simulink model "gm_lab2"  (R2022a)
settings: Solver=VariableStepAuto  StartTime=0.0  StopTime=5.0  RelTol=1e-3
settings Model: Creator=User  LastModifiedBy=User
settings OptimizationCC: BlockReduction=off  ConditionallyExecuteInputs=off
settings DebuggingCC: InheritedTsInSrcMsg=none

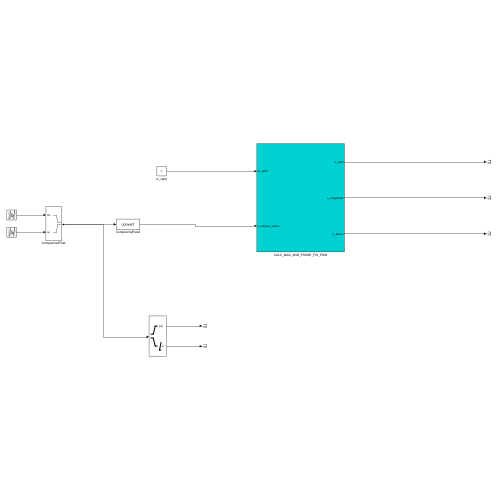
[thumbnail: Simulink's stored preview of the top-level diagram]
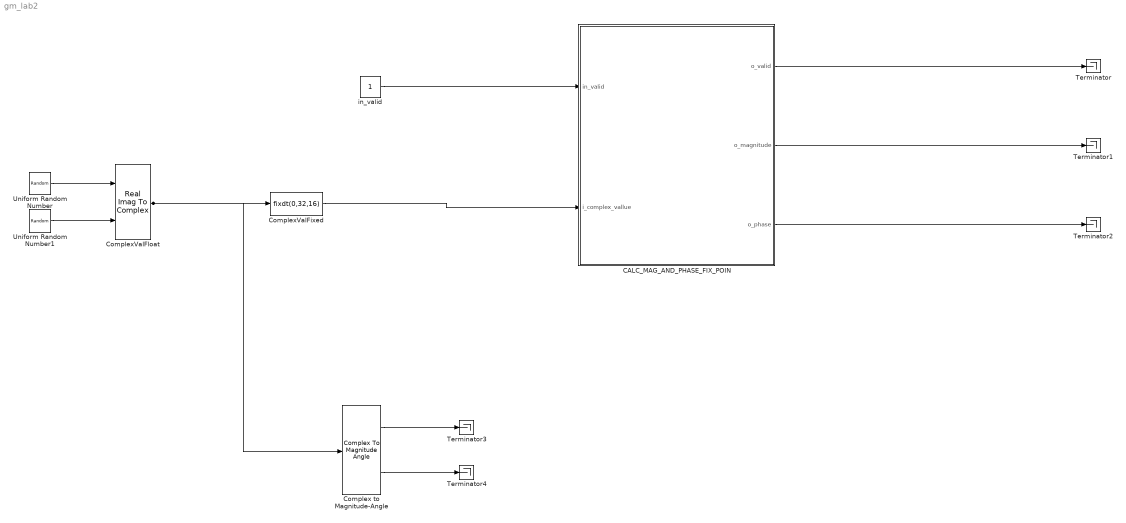
== system gm_lab2 ==
  CALC_MAG_AND_PHASE_FIX_POIN : Subsystem
  Complex to Magnitude-Angle : ComplexToMagnitudeAngle
  ComplexValFixed : DataTypeConversion  OutDataTypeStr=fixdt(0,32,16)  RndMeth=Round  SaturateOnIntegerOverflow=off
  ComplexValFloat : RealImagToComplex
  Terminator{,1..4} (5 alike) : Terminator
  Uniform Random Number : UniformRandomNumber  Minimum=0  Maximum=2 ^(16)-1  Seed=16  SampleTime=1
  Uniform Random Number1 : UniformRandomNumber  Minimum=0  Maximum=2 ^(16)-1  Seed=17  SampleTime=1
  in_valid : Constant  OutDataTypeStr=boolean  SampleTime=1
  wires:
  CALC_MAG_AND_PHASE_FIX_POIN/1(o_valid) -> Terminator/1
  in_valid/1 -> CALC_MAG_AND_PHASE_FIX_POIN/1(in_valid)
  CALC_MAG_AND_PHASE_FIX_POIN/3(o_phase) -> Terminator2/1
  CALC_MAG_AND_PHASE_FIX_POIN/2(o_magnitude) -> Terminator1/1
  ComplexValFixed/1 -> CALC_MAG_AND_PHASE_FIX_POIN/2(i_complex_vallue)
  Complex to Magnitude-Angle/2 -> Terminator4/1
  Complex to Magnitude-Angle/1 -> Terminator3/1
  ComplexValFloat/1 -> ComplexValFixed/1, Complex to Magnitude-Angle/1
  Uniform Random Number1/1 -> ComplexValFloat/2
  Uniform Random Number/1 -> ComplexValFloat/1

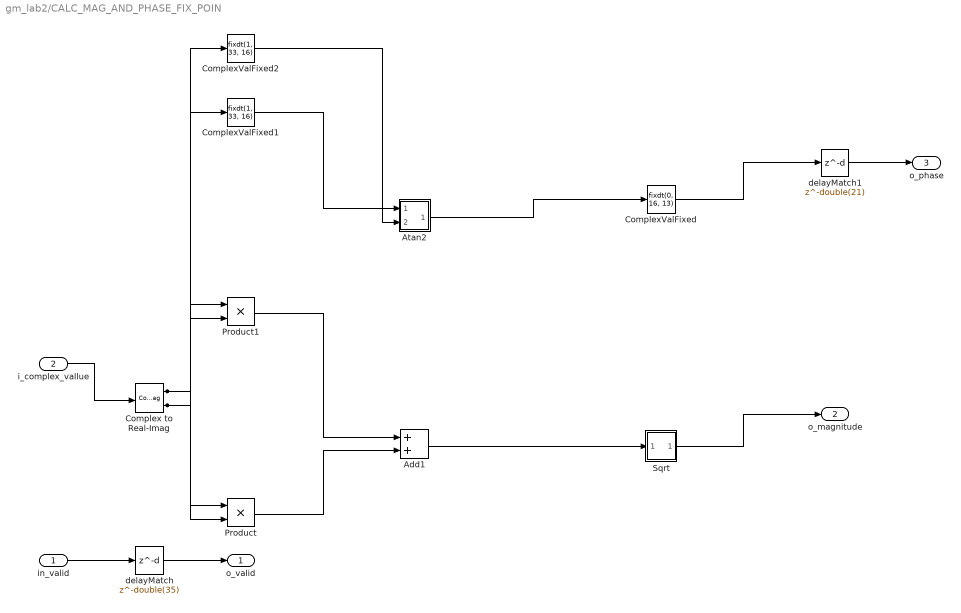
== system gm_lab2/CALC_MAG_AND_PHASE_FIX_POIN ==
  in_valid : Inport  OutDataTypeStr=boolean  PortDimensions=1  SampleTime=1
  i_complex_vallue : Inport  Port=2  OutDataTypeStr=fixdt(0, 32, 16)  PortDimensions=1  SampleTime=1
      settings: SignalType=complex
  Add1 : Sum  AccumDataTypeStr=fixdt(0, 65, 32)  OutDataTypeStr=fixdt(0, 65, 32)  SampleTime=1
  Atan2 : Subsystem
  Complex to Real-Imag : ComplexToRealImag  SampleTime=1
  ComplexValFixed : DataTypeConversion  OutDataTypeStr=fixdt(0, 16, 13)  RndMeth=Round  SampleTime=1  SaturateOnIntegerOverflow=off
  ComplexValFixed1 : DataTypeConversion  OutDataTypeStr=fixdt(1, 33, 16)  RndMeth=Round  SampleTime=1  SaturateOnIntegerOverflow=off
  ComplexValFixed2 : DataTypeConversion  OutDataTypeStr=fixdt(1, 33, 16)  RndMeth=Round  SampleTime=1  SaturateOnIntegerOverflow=off
  Product : Product  Inputs=**  OutDataTypeStr=fixdt(0, 64, 32)  SampleTime=1
  Product1 : Product  Inputs=**  OutDataTypeStr=fixdt(0, 64, 32)  SampleTime=1
  Sqrt : Subsystem
  delayMatch : Delay  DelayLength=double(35)  InitialCondition=0  SampleTime=1
  delayMatch1 : Delay  DelayLength=double(21)  InitialCondition=0  SampleTime=1
  o_valid : Outport  SampleTime=1
  o_magnitude : Outport  Port=2  SampleTime=1
  o_phase : Outport  Port=3  SampleTime=1
  wires:
  delayMatch/1 -> o_valid/1
  i_complex_vallue/1 -> Complex to Real-Imag/1
  Add1/1 -> Sqrt/1(In1)
  Atan2/1(Out1) -> ComplexValFixed/1
  Complex to Real-Imag/1 -> Product1/2, Product1/1, ComplexValFixed2/1
  Complex to Real-Imag/2 -> Product/2, Product/1, ComplexValFixed1/1
  delayMatch1/1 -> o_phase/1
  ComplexValFixed1/1 -> Atan2/1(In1)
  ComplexValFixed2/1 -> Atan2/2(In2)
  Product/1 -> Add1/2
  Product1/1 -> Add1/1
  Sqrt/1(Out1) -> o_magnitude/1
  in_valid/1 -> delayMatch/1
  ComplexValFixed/1 -> delayMatch1/1

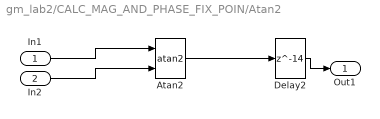
== system gm_lab2/CALC_MAG_AND_PHASE_FIX_POIN/Atan2 ==
  In1 : Inport
  In2 : Inport  Port=2
  Atan2 : Trigonometry  Operator=atan2  ApproximationMethod=CORDIC
  Delay2 : Delay  DelayLength=14
  Out1 : Outport
  wires:
  In1/1 -> Atan2/1
  In2/1 -> Atan2/2
  Atan2/1 -> Delay2/1
  Delay2/1 -> Out1/1

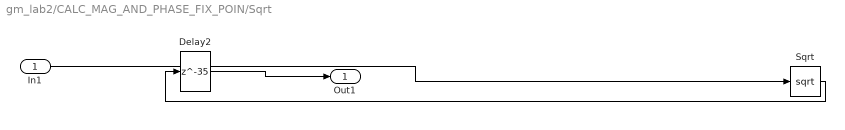
== system gm_lab2/CALC_MAG_AND_PHASE_FIX_POIN/Sqrt ==
  In1 : Inport
  Delay2 : Delay  DelayLength=35
  Sqrt : Sqrt  OutDataTypeStr=Inherit: Inherit via internal rule
  Out1 : Outport
  wires:
  In1/1 -> Sqrt/1
  Sqrt/1 -> Delay2/1
  Delay2/1 -> Out1/1
